simulink model "buckconverter"  (R2022b)
settings: Solver=VariableStepAuto  StartTime=0.0  StopTime=0.1  RelTol=1e-3
libraries: spsCurrentMeasurementLib x4, spsVoltageMeasurementLib x4, spsSeriesRLCBranchLib x3, spsMeanLib x3, spsDCVoltageSourceLib x1, spsDiodeLib x1, spsMosfetLib x1, sps_lib x1
settings Model: Creator=Zehra  LastModifiedBy=isild
settings OptimizationCC: ReuseModelBlockBuffer=on

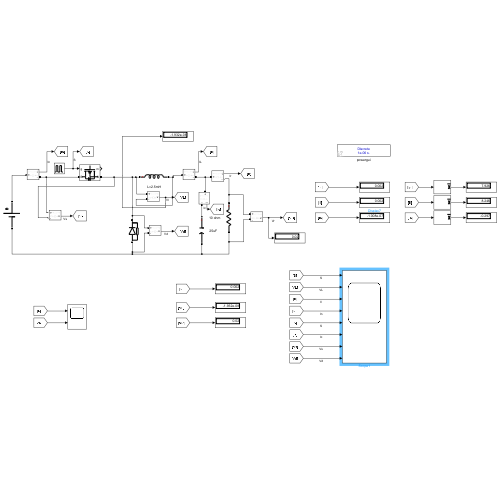
[thumbnail: Simulink's stored preview of the top-level diagram]
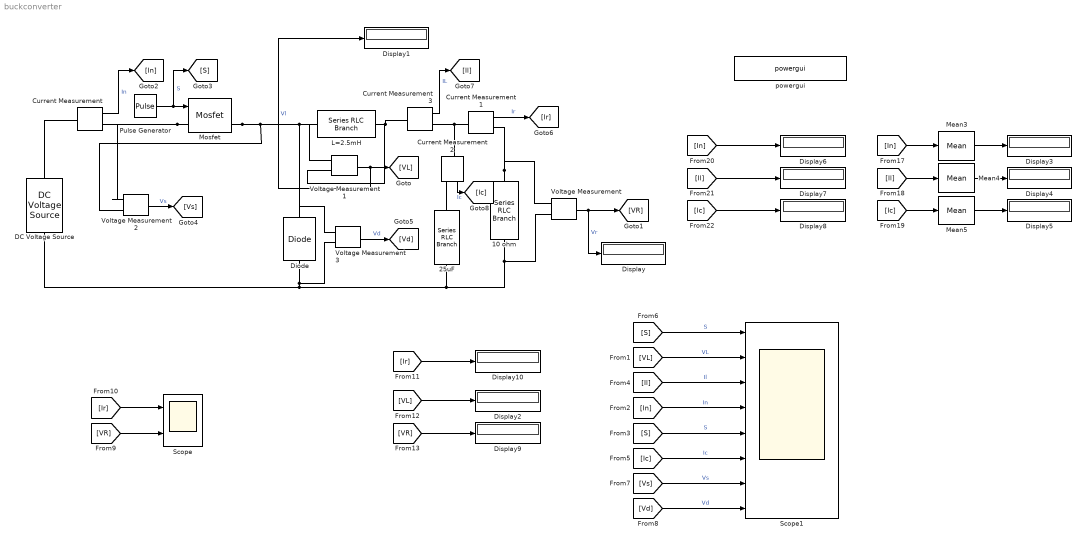
== system buckconverter ==
  10 ohm : spsSeriesRLCBranchLib/Series RLC Branch  LConnTagsString=__new0  RConnTagsString=__new0  BranchType=R  Resistance=10  Inductance=1e-3  SetiL0=off  InitialCurrent=0  Capacitance=1e-6  Setx0=off  InitialVoltage=0  Measurements=None
  25uF : spsSeriesRLCBranchLib/Series RLC Branch  LConnTagsString=__new0  RConnTagsString=__new0  BranchType=C  Resistance=20  Inductance=1e-3  SetiL0=off  InitialCurrent=0  Capacitance=25e-6  Setx0=off  InitialVoltage=0  Measurements=None
  Current Measurement{,1..3} (4 alike) : spsCurrentMeasurementLib/Current Measurement  PhasorSimulation=off  OutputType=Complex  PSBequivalent=0
  DC Voltage Source : spsDCVoltageSourceLib/DC Voltage Source  Amplitude=200  Measurements=None
  Diode : spsDiodeLib/Diode  Ron=0.001  Lon=0  Vf=0.8  IC=0  UseSnubber=0  Rs=500  Cs=250e-9  Measurements=off
  Display{,1..10} (11 alike) : Display
  L=2.5mH : spsSeriesRLCBranchLib/Series RLC Branch  LConnTagsString=__new0  RConnTagsString=__new0  BranchType=L  Resistance=20  Inductance=2.5e-3  SetiL0=off  InitialCurrent=0  Capacitance=100e-6  Setx0=off  InitialVoltage=0  Measurements=None
  Mean3 : spsMeanLib/Mean  Freq=60  Vinit=0  Ts=0
  Mean4 : spsMeanLib/Mean  Freq=60  Vinit=0  Ts=0
  Mean5 : spsMeanLib/Mean  Freq=60  Vinit=0  Ts=0
  Mosfet : spsMosfetLib/Mosfet  Ron=0.1  Lon=0  Rd=0.01  Vfd=0  IC=0  Rs=1e5  Cs=inf  Measurements=on
  Pulse Generator : DiscretePulseGenerator  PulseType=Time based  Period=1/100  PulseWidth=50
  Scope : Scope  NumInputPorts=2
  Scope1 : Scope  NumInputPorts=8
  Voltage Measurement{,1..3} (4 alike) : spsVoltageMeasurementLib/Voltage Measurement  PhasorSimulation=off  OutputType=Complex  PSBequivalent=0
  powergui : sps_lib/powergui  Priority=1  SimulationMode=Discrete  SampleTime=1e-6  frequency=60  Iterations=50  frequencyindice=0  Pbase=100e6  ErrMax=1e-4  UnitsV=kV  UnitsW=MW  buscounter=0  FunctionMessages=off  echomessages=off  EnableUseOfTLC=off  CurrentSourceSwitches=off  DisableSnubberDevices=off  DisableRonSwitches=off  DisableVfSwitches=off  DisplayEquations=off  AutomaticDiscreteSolvers=off  SolverType=Tustin/Backward Euler (TBE)  Interpol=off  ExternalGateDelay=off  methode=off  Ts=100  x0status=blocks  SPID=on  SwTol=0  HookPort=off  NonlinearTolerance=1e-4  nMaxIteration=100  ContinueOnMaxIteration=off  RestoreLinks=warning  ResistiveCurrentMeasurement=off  Frange=[0:2:500]  Ylog=off  Xlog=on  ShowGrid=off  save=off  variable=ZData  structure=0  ZoomFFT=off  StartTime=0.0  cycles=1  DisplayStyle=1  fundamental=60  FreqAxis=off  MaxFrequency=1000  frequencyindicesteady=1  RmsSteady=1  display=off
  wires:
  Voltage Measurement2/1 -> [Vs]  "Vs"
  Pulse Generator/1 -> [S], Mosfet/1  "S"
  Current Measurement/1 -> [In]  "In"
  Voltage Measurement/1 -> Display/1, [VR]  "Vr"
  Voltage Measurement3/1 -> [Vd]  "Vd"
  Current Measurement1/1 -> [Ir]  "Ir"
  Current Measurement3/1 -> [Il]  "IL"
  Current Measurement2/1 -> [Ic]  "Ic"
  [S] -> Scope1/1  "S"
  [VL] -> Scope1/2  "VL"
  [S] -> Scope1/5  "S"
  [In] -> Scope1/4  "In"
  [Il] -> Scope1/3  "Il"
  [Vd] -> Scope1/8  "Vd"
  [Vs] -> Scope1/7  "Vs"
  [Ic] -> Scope1/6  "Ic"
  [Ir] -> Scope/1
  [VR] -> Scope/2
  Voltage Measurement1/1 -> Display1/1, [VL]  "Vl"
  Mean5/1 -> Display5/1
  [Il] -> Display7/1
  [Ic] -> Mean5/1
  [Ic] -> Display8/1
  [In] -> Display6/1
  Mean4/1 -> Display4/1
  Mean3/1 -> Display3/1
  [Il] -> Mean4/1
  [In] -> Mean3/1
  [Ir] -> Display10/1
  [VL] -> Display2/1
  [VR] -> Display9/1
  connections:
  Mosfet/RConn1 -- Voltage Measurement3/LConn1 -- Diode/RConn1 -- Voltage Measurement1/LConn1 -- L=2.5mH/LConn1 -- Voltage Measurement2/LConn2
  Voltage Measurement1/LConn2 -- Current Measurement3/LConn1 -- L=2.5mH/RConn1
  Diode/LConn1 -- Voltage Measurement3/LConn2 -- DC Voltage Source/LConn1 -- 25uF/RConn1 -- Voltage Measurement/LConn2 -- 10 ohm/RConn1
  10 ohm/LConn1 -- Voltage Measurement/LConn1 -- Current Measurement1/RConn1
  Mosfet/LConn1 -- Voltage Measurement2/LConn1 -- Current Measurement/RConn1
  Current Measurement/LConn1 -- DC Voltage Source/RConn1
  Current Measurement3/RConn1 -- Current Measurement2/LConn1 -- Current Measurement1/LConn1
  Current Measurement2/RConn1 -- 25uF/LConn1
